simulink model "VSC_GF_linear_4_pu"  (R2020a)
settings: Solver=ode3  StartTime=0.0  StopTime=Tsim  FixedStep=10e-6  RelTol=1e-5  EnableMultiTasking=on
values from neighbouring files (symbols this model uses):
  Afdroop_n1 = [-1/tau_droop_f]    [linear_model_pu.m]
  Aig_n1 = [-R_pcc/L_pcc -wb_n1 ... (first row only)    [linear_model_pu.m]
  Ais_n1 = [0 0 ... (first row only)    [linear_model_pu.m]
  Alc_n1 = [(-Rc_n1-Rac_n1)/Lc_n1 -wb_n1 -1/Lc_n1 0 ... (first row only)    [linear_model_pu.m]
  angle_g1_fnl = 0.0    (= 0)    [params_pu.m]
  angle_g1_init = 0.0    (= 0)    [params_pu.m]
  Atheta_n1 = [0]    [linear_model_pu.m]
  Au_n1 = [0 0 ... (first row only)    [linear_model_pu.m]
  Audroop_n1 = [-1/tau_droop_u]    [linear_model_pu.m]
  Avgc_n1 = [0]    [linear_model_pu.m]
  Awc_n1 = [0]    [linear_model_pu.m]
  Awg_g1 = [0]    [linear_model_pu.m]
  Bfdroop_n1 = [0 3*ig_q0_n1/2 3*ig_d0_n1/2 3*u_q0_n1/2 3*u_d0_n1/2]    [linear_model_pu.m]
  Big_n1 = [-1/L_pcc 0 1/L_pcc 0 -ig_d0_n1 ... (first row only)    [linear_model_pu.m]
  Bis_n1 = [1 0 -1 0 0 0 ... (first row only)    [linear_model_pu.m]
  Blc_n1 = [1/Lc_n1 0 Rac_n1/Lc_n1 0 -is_d0_n1 ... (first row only)    [linear_model_pu.m]
  Btheta_n1 = [0 0]    [linear_model_pu.m]
  Bu_n1 = [1 0 -1 0 0 0 ... (first row only)    [linear_model_pu.m]
  Budroop_n1 = [0 -3*ig_d0_n1/2 3*ig_q0_n1/2 3*u_d0_n1/2 -3*u_q0_n1/2]    [linear_model_pu.m]
  Bvgc_n1 = [0 0 0]    [linear_model_pu.m]
  Bwc_n1 = [1]    [linear_model_pu.m]
  Bwg_g1 = [1 0]    [linear_model_pu.m]
  Cfdroop_n1 = [-k_droop_f_n1/tau_droop_f*wb_n1]    [linear_model_pu.m]
  Cig_n1 = [1 0 ... (first row only)    [linear_model_pu.m]
  Cis_n1 = [+ki_s_n1 0 ... (first row only)    [linear_model_pu.m]
  Clc_n1 = [1 0 0 0 ... (first row only)    [linear_model_pu.m]
  Ctheta_n1 = [0]    [linear_model_pu.m]
  Cu_n1 = [+ki_vac_n1 0 ... (first row only)    [linear_model_pu.m]
  Cudroop_n1 = [k_droop_u_n1/tau_droop_u]    [linear_model_pu.m]
  Cvgc_n1 = [0 ... (first row only)    [linear_model_pu.m]
  Cwc_n1 = [1]    [linear_model_pu.m]
  Cwg_g1 = [1]    [linear_model_pu.m]
  Dfdroop_n1 = [+k_droop_f_n1*wb_n1 0 0 0 0]    [linear_model_pu.m]
  Dig_n1 = [0 0 0 0 0 ... (first row only)    [linear_model_pu.m]
  Dis_n1 = [+kp_s_n1 0 -kp_s_n1 +wb_n1*Lc_n1 1 0 ... (first row only)    [linear_model_pu.m]
  Dlc_n1 = [0 0 0 0 0 ... (first row only)    [linear_model_pu.m]
  Dtheta_n1 = [1 -1]    [linear_model_pu.m]
  Du_n1 = [+kp_vac_n1 0 -kp_vac_n1 +wb_n1*Cac_n1 1 0 ... (first row only)    [linear_model_pu.m]
  Dudroop_n1 = [+k_droop_u_n1 0 0 0 0]    [linear_model_pu.m]
  Dvgc_n1 = [cos(etheta0) -sin(etheta0) -sin(etheta0)*vg_q0_n1-cos(etheta0)*vg_d0_n1 ... (first row only)    [linear_model_pu.m]
  Dwc_n1 = [0]    [linear_model_pu.m]
  Dwg_g1 = [0 1]    [linear_model_pu.m]
  f1_0 = freq_real_n1_pu(index0)    [linear_model_pu.m]
  ig_dc0_n1 = igc_d_real_n1_pu(index0)    [linear_model_pu.m]
  ig_qc0_n1 = igc_q_real_n1_pu(index0)    [linear_model_pu.m]
  is_dc0_n1 = is_d_real_n1_pu(index0)    [linear_model_pu.m]
  is_qc0_n1 = is_q_real_n1_pu(index0)    [linear_model_pu.m]
  magnitud_delay = 1e-5    (= 1e-05)    [params_pu.m]
  plots_step = 10e-6    (= 1e-05)    [params_pu.m]
  T_stp = Tsim/2    (= 2)    [params_pu.m]
  u_dc0_n1 = u_d_real_n1_pu(index0)    [linear_model_pu.m]
  u_qc0_n1 = u_q_real_n1_pu(index0)    [linear_model_pu.m]
  vc_dc0_n1 = vc_d_real_n1_pu(index0)    [linear_model_pu.m]
  vc_qc0_n1 = vc_q_real_n1_pu(index0)    [linear_model_pu.m]
  Vpeak_g1_fnl = 0.98*(sqrt(2)/sqrt(3))    [params_pu.m]
  Vpeak_g1_init = 1*(sqrt(2)/sqrt(3))    [params_pu.m]
undefined symbols (not defined in the file or in its folder): Af_ig, Af_u, Bf_ig, Bf_u, Cf_ig, Cf_u, Df_ig, Df_u
libraries: cstblocks x1
settings Model: Creator=Agustí  LastModifiedBy=Saman
settings SolverCC: ZeroCrossAlgorithm=Adaptive
settings DataIOCC: LimitDataPoints=on  SaveFormat=Array  SignalLoggingSaveFormat=ModelDataLogs  ReturnWorkspaceOutputs=off
settings OptimizationCC: BlockReduction=off  BufferReuse=off  ExpressionDepthLimit=2147483647  LifeSpan=inf
settings DebuggingCC: AlgebraicLoopMsg=none  UnderspecifiedInitializationDetection=Classic  MergeDetectMultiDrivingBlocksExec=none  FcnCallInpInsideContextMsg=warning  UnconnectedInputMsg=none  UnconnectedOutputMsg=none  UnconnectedLineMsg=none  AllowSymbolicDim=off  StateNameClashWarn=warning  SFUnexpectedBacktrackingDiag=warning  SFNoUnconditionalDefaultTransitionDiag=warning  SFExecutionAtInitializationDiag=none  ArithmeticOperatorsInVariantConditions=warning
settings HardwareCC: ProdBitPerPointer=32  ProdBitPerSizeT=32  ProdBitPerPtrDiffT=32  ProdLargestAtomicFloat=None  ProdIntDivRoundTo=Undefined  ProdEndianess=Unspecified  ProdWordSize=32  ProdHWDeviceType=32-bit Generic
settings ModelReferenceCC: PropagateSignalLabelsOutOfModel=off
settings SFSimCC: SimUseLocalCustomCode=off  CustomCodeUndefinedFunction=UseInterfaceOnly
settings RTWCC: RTWUseLocalCustomCode=off
settings CodeAppCC: StateflowObjectComments=on
settings GRTTargetCC: TargetLangStandard=C89/C90 (ANSI)
settings ConfigComp: CovMetricSettings=dw  CovHtmlReporting=on  CovSaveCumulativeToWorkspaceVar=on  CovSaveSingleToWorkspaceVar=on  CovExternalEMLEnable=off  CovSFcnEnable=off
settings SimscapeCC: SimscapeNormalizeSystem=off
settings ConfigurationSet: Description=SimMechanics 2G

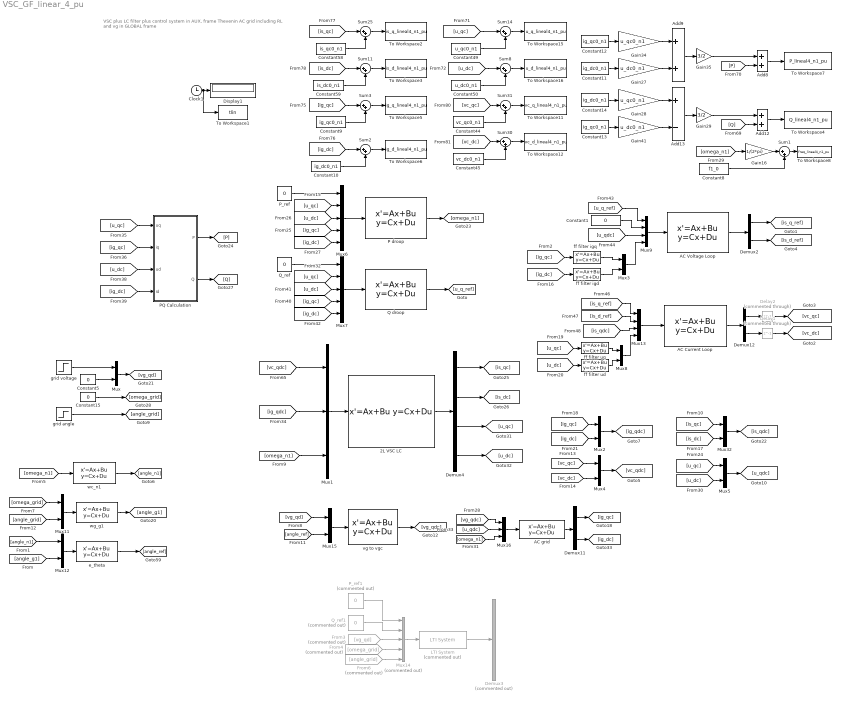
== system VSC_GF_linear_4_pu ==
  note: VSC plus LC filter plus control system in AUX. frame
      |
      | Thevenin AC grid including RL and vg in GLOBAL frame
  2L VSC LC : StateSpace  A=Alc_n1  B=Blc_n1  C=Clc_n1  D=Dlc_n1  InitialCondition=[0 0 0 0]
  AC Current Loop : StateSpace  A=Ais_n1  B=Bis_n1  C=Cis_n1  D=Dis_n1  InitialCondition=[0 0]
  AC Voltage Loop : StateSpace  A=Au_n1  B=Bu_n1  C=Cu_n1  D=Du_n1  InitialCondition=[0 0]
  AC grid : StateSpace  A=Aig_n1  B=Big_n1  C=Cig_n1  D=Dig_n1  InitialCondition=[0]
  Add12 : Sum
  Add13 : Sum  Inputs=+-
  Add8 : Sum
  Add9 : Sum
  Clock1 : Clock
  Constant1 : Constant  Value=0
  Constant10 : Constant  Value=ig_dc0_n1
  Constant11 : Constant  Value=ig_dc0_n1
  Constant12 : Constant  Value=ig_qc0_n1
  Constant13 : Constant  Value=ig_qc0_n1
  Constant14 : Constant  Value=ig_dc0_n1
  Constant15 : Constant  Value=0
  Constant44 : Constant  Value=vc_qc0_n1
  Constant45 : Constant  Value=vc_dc0_n1
  Constant49 : Constant  Value=u_qc0_n1
  Constant5 : Constant  Value=0
  Constant50 : Constant  Value=u_dc0_n1
  Constant58 : Constant  Value=is_qc0_n1
  Constant59 : Constant  Value=is_dc0_n1
  Constant8 : Constant  Value=f1_0
  Constant9 : Constant  Value=ig_qc0_n1
  Delay1 : Delay  Commented=through  DelayLength=1  InitialCondition=0  SampleTime=magnitud_delay
  Delay2 : Delay  Commented=through  DelayLength=1  InitialCondition=0  SampleTime=magnitud_delay
  Demux11 : Demux  Outputs=2
  Demux12 : Demux  Outputs=2
  Demux2 : Demux  Outputs=2
  Demux3 : Demux  Commented=on  Outputs=8
  Demux4 : Demux
  Display1 : Display
  From3 : From  Commented=on  GotoTag=vg_qd
  From4 : From  Commented=on  GotoTag=omega_grid
  From6 : From  Commented=on  GotoTag=angle_grid
  Gain16 : Gain  Gain=1/(2*pi)
  Gain27 : Gain  Gain=u_dc0_n1
  Gain28 : Gain  Gain=u_qc0_n1
  Gain29 : Gain  Gain=3/2
  Gain34 : Gain  Gain=u_qc0_n1
  Gain35 : Gain  Gain=3/2
  Gain41 : Gain  Gain=u_dc0_n1
  LTI System : cstblocks/LTI System  Commented=on  sys=ss_vsc  IC=zeros(1,15)
  Mux{,2..5,8,11..12,15,32} (10 alike) : Mux  Inputs=2
  Mux1 : Mux  Inputs=3
  Mux13 : Mux
  Mux14 : Mux  Commented=on  Inputs=5
  Mux16 : Mux  Inputs=3
  Mux6 : Mux  Inputs=5
  Mux7 : Mux  Inputs=5
  Mux9 : Mux
  P droop : StateSpace  A=Afdroop_n1  B=Bfdroop_n1  C=Cfdroop_n1  D=Dfdroop_n1  InitialCondition=[0]
  PQ Calculation : Subsystem
  P_ref : Constant  Value=0
  P_ref1 : Constant  Commented=on  Value=0
  Q droop : StateSpace  A=Audroop_n1  B=Budroop_n1  C=Cudroop_n1  D=Dudroop_n1  InitialCondition=[0]
  Q_ref : Constant  Value=0
  Q_ref1 : Constant  Commented=on  Value=0
  Sum{1..3,8,11,14,25,30..31} (9 alike) : Sum  Inputs=|++
  To Workspace1 : ToWorkspace  VariableName=tlin  SampleTime=plots_step
  To Workspace11 : ToWorkspace  VariableName=vc_q_lineal4_n1_pu  SampleTime=plots_step
  To Workspace12 : ToWorkspace  VariableName=vc_d_lineal4_n1_pu  SampleTime=plots_step
  To Workspace15 : ToWorkspace  VariableName=u_q_lineal4_n1_pu  SampleTime=plots_step
  To Workspace16 : ToWorkspace  VariableName=u_d_lineal4_n1_pu  SampleTime=plots_step
  To Workspace2 : ToWorkspace  VariableName=is_q_lineal4_n1_pu  SampleTime=plots_step
  To Workspace3 : ToWorkspace  VariableName=is_d_lineal4_n1_pu  SampleTime=plots_step
  To Workspace4 : ToWorkspace  VariableName=Q_lineal4_n1_pu  SampleTime=plots_step
  To Workspace5 : ToWorkspace  VariableName=ig_q_lineal4_n1_pu  SampleTime=plots_step
  To Workspace6 : ToWorkspace  VariableName=ig_d_lineal4_n1_pu  SampleTime=plots_step
  To Workspace7 : ToWorkspace  VariableName=P_lineal4_n1_pu  SampleTime=plots_step
  To Workspace8 : ToWorkspace  VariableName=freq_lineal4_n1_pu  SampleTime=plots_step
  e_theta : StateSpace  A=Atheta_n1  B=Btheta_n1  C=Ctheta_n1  D=Dtheta_n1  InitialCondition=[0]
  ff filter igd : StateSpace  A=Af_ig  B=Bf_ig  C=Cf_ig  D=Df_ig  InitialCondition=[0]
  ff filter igq : StateSpace  A=Af_ig  B=Bf_ig  C=Cf_ig  D=Df_ig  InitialCondition=[0]
  ff filter ud : StateSpace  A=Af_u  B=Bf_u  C=Cf_u  D=Df_u  InitialCondition=[0]
  ff filter uq : StateSpace  A=Af_u  B=Bf_u  C=Cf_u  D=Df_u  InitialCondition=[0]
  grid angle : Step  Time=T_stp  Before=angle_g1_init  After=angle_g1_fnl  SampleTime=0
  grid voltage : Step  Time=T_stp  Before=Vpeak_g1_init-1*(sqrt(2)/sqrt(3))  After=Vpeak_g1_fnl-1*(sqrt(2)/sqrt(3))  SampleTime=0
  vg to vgc : StateSpace  A=Avgc_n1  B=Bvgc_n1  C=Cvgc_n1  D=Dvgc_n1  InitialCondition=[0]
  wc_n1 : StateSpace  A=Awc_n1  B=Bwc_n1  C=Cwc_n1  D=Dwc_n1  InitialCondition=[0]
  wg_g1 : StateSpace  A=Awg_g1  B=Bwg_g1  C=Cwg_g1  D=Dwg_g1  InitialCondition=[0]
  wires:
  Clock1/1 -> To Workspace1/1, Display1/1
  [omega_n1] -> wc_n1/1
  PQ Calculation/2(Q) -> [Q]
  [ig_dc] -> PQ Calculation/4(id)
  wc_n1/1 -> [angle_n1]
  [vc_qc] -> Mux4/1
  [u_qc] -> PQ Calculation/1(uq)
  Mux4/1 -> [vc_qdc]
  [vc_dc] -> Mux4/2
  [ig_qc] -> PQ Calculation/2(iq)
  Add8/1 -> To Workspace7/1
  Sum25/1 -> To Workspace2/1
  PQ Calculation/1(P) -> [P]
  grid voltage/1 -> Mux/1
  2L VSC LC/1 -> Demux4/1
  Mux/1 -> [vg_qd]
  Constant58/1 -> Sum25/2
  Constant10/1 -> Sum2/2
  [u_dc] -> Sum8/1
  Constant9/1 -> Sum3/2
  Mux5/1 -> [u_qdc]
  [u_qc] -> Mux5/1
  [u_dc] -> PQ Calculation/3(ud)
  [u_dc] -> Mux5/2
  [ig_dc] -> Mux2/2
  [is_dc] -> Mux32/2
  Sum11/1 -> To Workspace3/1
  [is_qc] -> Sum25/1
  grid angle/1 -> [angle_grid]
  Sum8/1 -> To Workspace16/1
  Sum31/1 -> To Workspace11/1
  Demux4/2 -> [is_dc]
  [u_qc] -> Sum14/1
  Constant45/1 -> Sum30/2
  Mux32/1 -> [is_qdc]
  Gain41/1 -> Add13/2
  Constant44/1 -> Sum31/2
  Constant49/1 -> Sum14/2
  [is_qc] -> Mux32/1
  Gain35/1 -> Add8/1
  [vc_dc] -> Sum30/1
  Gain28/1 -> Add13/1
  Constant5/1 -> Mux/2
  Constant14/1 -> Gain28/1
  Constant50/1 -> Sum8/2
  Constant15/1 -> [omega_grid]
  Sum30/1 -> To Workspace12/1
  [ig_qc] -> Mux2/1
  Constant12/1 -> Gain34/1
  Demux4/1 -> [is_qc]
  [is_dc] -> Sum11/1
  Sum3/1 -> To Workspace5/1
  Demux4/4 -> [u_dc]
  Add9/1 -> Gain35/1
  Add13/1 -> Gain29/1
  [vc_qc] -> Sum31/1
  Gain29/1 -> Add12/1
  Gain27/1 -> Add9/2
  Gain34/1 -> Add9/1
  [omega_n1] -> Mux1/3
  Demux4/3 -> [u_qc]
  [P] -> Add8/2
  [Q] -> Add12/2
  [ig_dc] -> Sum2/1
  [vc_qdc] -> Mux1/1
  Add12/1 -> To Workspace4/1
  [ig_qc] -> Sum3/1
  Sum2/1 -> To Workspace6/1
  Constant13/1 -> Gain41/1
  Sum14/1 -> To Workspace15/1
  Constant59/1 -> Sum11/2
  Mux1/1 -> 2L VSC LC/1
  [ig_qdc] -> Mux1/2
  Constant11/1 -> Gain27/1
  Mux2/1 -> [ig_qdc]
  Mux6/1 -> P droop/1
  [u_qc] -> Mux6/2
  [u_dc] -> Mux6/3
  [ig_qc] -> Mux6/4
  [ig_dc] -> Mux6/5
  P_ref/1 -> Mux6/1
  P droop/1 -> [omega_n1]
  [omega_n1] -> Gain16/1
  Sum1/1 -> To Workspace8/1
  Gain16/1 -> Sum1/1
  Constant8/1 -> Sum1/2
  Q droop/1 -> [u_q_ref]
  [u_qc] -> Mux7/2
  Q_ref/1 -> Mux7/1
  [ig_qc] -> Mux7/4
  [u_dc] -> Mux7/3
  [ig_dc] -> Mux7/5
  Mux7/1 -> Q droop/1
  Constant1/1 -> Mux9/2
  Mux9/1 -> AC Voltage Loop/1
  [u_q_ref] -> Mux9/1
  [u_qdc] -> Mux9/3
  Mux3/1 -> Mux9/4
  AC Voltage Loop/1 -> Demux2/1
  Demux2/1 -> [is_q_ref]
  Demux2/2 -> [is_d_ref]
  Mux13/1 -> AC Current Loop/1
  [is_q_ref] -> Mux13/1
  [is_d_ref] -> Mux13/2
  [is_qdc] -> Mux13/3
  Mux8/1 -> Mux13/4
  Demux12/2 -> Delay1/1
  AC Current Loop/1 -> Demux12/1
  Demux12/1 -> Delay2/1
  Delay1/1 -> [vc_dc]
  Delay2/1 -> [vc_qc]
  Mux11/1 -> wg_g1/1
  [omega_grid] -> Mux11/1
  [angle_grid] -> Mux11/2
  wg_g1/1 -> [angle_g1]
  Mux12/1 -> e_theta/1
  [angle_g1] -> Mux12/2
  [angle_n1] -> Mux12/1
  e_theta/1 -> [angle_ref]
  Mux14/1 -> LTI System/1
  LTI System/1 -> Demux3/1
  From6/1 -> Mux14/5
  From4/1 -> Mux14/4
  From3/1 -> Mux14/3
  P_ref1/1 -> Mux14/1
  Q_ref1/1 -> Mux14/2
  Mux16/1 -> AC grid/1
  Demux11/1 -> [ig_qc]
  [vg_qd] -> Mux15/1
  Demux11/2 -> [ig_dc]
  vg to vgc/1 -> [vg_qdc]
  AC grid/1 -> Demux11/1
  [angle_ref] -> Mux15/2
  [vg_qdc] -> Mux16/1
  [u_qdc] -> Mux16/2
  Mux15/1 -> vg to vgc/1
  [omega_n1] -> Mux16/3
  [ig_qc] -> ff filter igq/1
  [ig_dc] -> ff filter igd/1
  ff filter igq/1 -> Mux3/1
  ff filter igd/1 -> Mux3/2
  ff filter uq/1 -> Mux8/1
  ff filter ud/1 -> Mux8/2
  [u_qc] -> ff filter uq/1
  [u_dc] -> ff filter ud/1

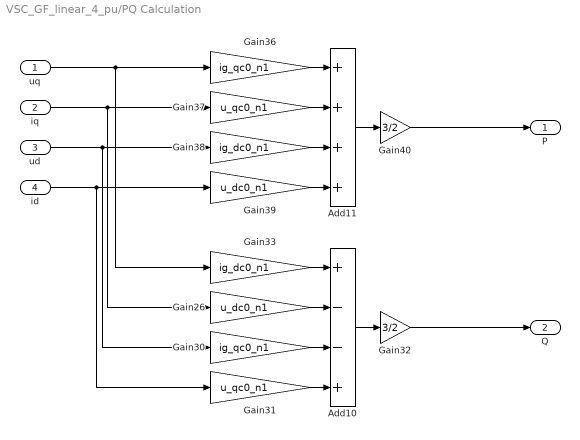
== system VSC_GF_linear_4_pu/PQ Calculation ==
  uq : Inport
  iq : Inport  Port=2
  ud : Inport  Port=3
  id : Inport  Port=4
  Add10 : Sum  Inputs=+--+
  Add11 : Sum  Inputs=++++
  Gain26 : Gain  Gain=u_dc0_n1
  Gain30 : Gain  Gain=ig_qc0_n1
  Gain31 : Gain  Gain=u_qc0_n1
  Gain32 : Gain  Gain=3/2
  Gain33 : Gain  Gain=ig_dc0_n1
  Gain36 : Gain  Gain=ig_qc0_n1
  Gain37 : Gain  Gain=u_qc0_n1
  Gain38 : Gain  Gain=ig_dc0_n1
  Gain39 : Gain  Gain=u_dc0_n1
  Gain40 : Gain  Gain=3/2
  P : Outport
  Q : Outport  Port=2
  wires:
  Gain39/1 -> Add11/4
  Add10/1 -> Gain32/1
  Gain40/1 -> P/1
  Gain31/1 -> Add10/4
  Gain36/1 -> Add11/1
  Gain26/1 -> Add10/2
  Gain30/1 -> Add10/3
  Gain38/1 -> Add11/3
  id/1 -> Gain31/1, Gain39/1
  Gain37/1 -> Add11/2
  Add11/1 -> Gain40/1
  Gain33/1 -> Add10/1
  ud/1 -> Gain30/1, Gain38/1
  iq/1 -> Gain26/1, Gain37/1
  uq/1 -> Gain33/1, Gain36/1
  Gain32/1 -> Q/1
